simulink model "Task_8"  (R2016b)
settings: Solver=VariableStepAuto  StartTime=0.0  StopTime=10.0  RelTol=1e-5
undefined symbols (not defined in the file or in its folder): K
settings Model: Creator=Suvansh  LastModifiedBy=Suvansh
settings SolverCC: MaxConsecutiveMinStep=10

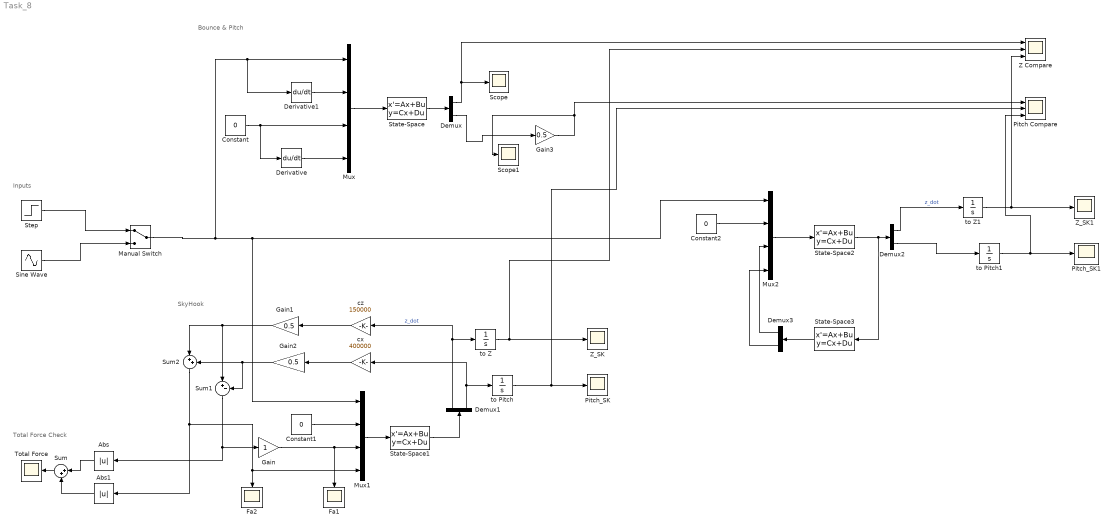
== system Task_8 ==
  note: Inputs
  note: Total Force Check
  note: SkyHook
  note: Bounce & Pitch
  Abs : Abs
  Abs1 : Abs
  Constant : Constant  Value=0
  Constant1 : Constant  Value=0
  Constant2 : Constant  Value=0
  Demux{,1..3} (4 alike) : Demux  Outputs=2
  Derivative : Derivative
  Derivative1 : Derivative
  Fa1 : Scope
  Fa2 : Scope
  Gain : Gain
  Gain1 : Gain  Gain=0.5
  Gain2 : Gain  Gain=0.5
  Gain3 : Gain  Gain=0.5
  Manual Switch : ManualSwitch
  Mux : Mux
  Mux1 : Mux
  Mux2 : Mux
  Pitch Compare : Scope  NumInputPorts=3
  Pitch_SK : Scope
  Pitch_SK1 : Scope
  Scope : Scope
  Scope1 : Scope
  Sine Wave : Sin  Amplitude=0.01  Frequency=6.28  SampleTime=0
  State-Space : StateSpace  A=[0 1 0 0 ; (k1 + k2)*(-1/m) (c1 + c2)*(-1/m) ((1-Lambda)*k2 -Lambda*k1)*(-L/m) ((1-Lambda)*c2 - Lambda*c1)*(-L/m); 0 0 0 1; ((1-Lambda)*k2 - Lambda*k1)*(-L/j) ((1-Lambda)*c2 - Lambda*c1)*(-L/j) (Lambda*Lambda*k1 + (1- Lambda)*(1-Lambda)*k2)*(-(L*L)/j) (Lambda*Lambda*c1 + (1- Lambda)*(1-Lambda)*c2)*(-(L*L)/j )] ;  B=|  C=[1 0 0 0; 0 0 1 0;]  D=[0 0 0 0;0 0 0 0]  X0=0
      | [  0 0 0 0; k1/m c1/m k2/m c2/m ;      0 0 0 0; 
      |      (-k1*Lambda*L)/j (-c1*Lambda*L)/j (k2*(1-Lambda)*L)/j (c2*(1-Lambda)*L)/j;
      | 
      | ] ;
  State-Space1 : StateSpace  A=|  B=|  C=|  D=[ 0 0 0 0 ; 0 0 0 0;];  X0=0
      A=|
      | [0 1 0 0
      |  ;  -2*k/m 0 0 0
      |  ;   0 0 0 1
      |  ;   0 0 -2*k*L^2/j 0];
      B=|
      | [0 0 0 0
      |   ;  k/m k/m -1/m -1/m
      |  ;   0 0 0 0
      |    ; -L*k/j L*k/j L/j -L/j];
      C=|
      | [0 1 0 0
      |     0 0 0 1];
  State-Space2 : StateSpace  A=|  B=|  C=|  D=[ 0 0 0 0 ; 0 0 0 0;];  X0=0
      A=|
      | [0 1 0 0
      |  ;  -2*k/m 0 0 0
      |  ;   0 0 0 1
      |  ;   0 0 -2*k*L^2/j 0];
      B=|
      | [0 0 0 0
      |   ;  k/m k/m -1/m -1/m
      |  ;   0 0 0 0
      |    ; -L*k/j L*k/j L/j -L/j];
      C=|
      | [0 1 0 0
      |     0 0 0 1];
  State-Space3 : StateSpace  A=K.A  B=K.B  C=K.C  D=K.D  X0=0
  Step : Step  After=0.03  SampleTime=0
  Sum : Sum  Inputs=|++
  Sum1 : Sum  Inputs=|+-
  Sum2 : Sum  Inputs=|++
  Total Force : Scope
  Z Compare : Scope  NumInputPorts=3
  Z_SK : Scope
  Z_SK1 : Scope
  cx : Gain  Gain=400000
  cz : Gain  Gain=150000
  to Pitch : Integrator
  to Pitch1 : Integrator
  to Z : Integrator
  to Z1 : Integrator
  wires:
  Derivative/1 -> Mux/4
  Mux/1 -> State-Space/1
  Demux/2 -> Gain3/1
  Demux/1 -> Scope/1, Z Compare/1
  Constant/1 -> Derivative/1, Mux/3
  State-Space/1 -> Demux/1
  Derivative1/1 -> Mux/2
  Mux1/1 -> State-Space1/1
  Manual Switch/1 -> Derivative1/1, Mux/1, Mux2/1, Mux1/1
  Constant1/1 -> Mux1/2
  State-Space1/1 -> Demux1/1
  Demux1/1 -> cz/1, to Z/1  "z_dot"
  Demux1/2 -> cx/1, to Pitch/1
  cx/1 -> Gain2/1
  cz/1 -> Gain1/1
  Sum2/1 -> Abs1/1, Fa2/1, Mux1/4
  Gain2/1 -> Sum2/2, Sum1/2
  Gain1/1 -> Sum2/1, Sum1/1
  Sum1/1 -> Gain/1, Abs/1
  Abs/1 -> Sum/1
  Abs1/1 -> Sum/2
  Sum/1 -> Total Force/1
  to Z/1 -> Z Compare/2, Z_SK/1
  to Pitch/1 -> Pitch_SK/1, Pitch Compare/2
  Gain/1 -> Mux1/3, Fa1/1
  Sine Wave/1 -> Manual Switch/2
  Step/1 -> Manual Switch/1
  Gain3/1 -> Scope1/1, Pitch Compare/1
  Mux2/1 -> State-Space2/1
  Constant2/1 -> Mux2/2
  State-Space2/1 -> State-Space3/1, Demux2/1
  Demux2/1 -> to Z1/1  "z_dot"
  Demux2/2 -> to Pitch1/1
  to Z1/1 -> Z Compare/3, Z_SK1/1
  to Pitch1/1 -> Pitch Compare/3, Pitch_SK1/1
  State-Space3/1 -> Demux3/1
  Demux3/1 -> Mux2/3
  Demux3/2 -> Mux2/4
